simulink model "problem1"  (R2020b)
settings: Solver=VariableStepAuto  StartTime=0.0  StopTime=10.0  RelTol=1e-3
undefined symbols (not defined in the file): b, K1, K12, M1, M2
settings Model: Creator=admin  LastModifiedBy=admin

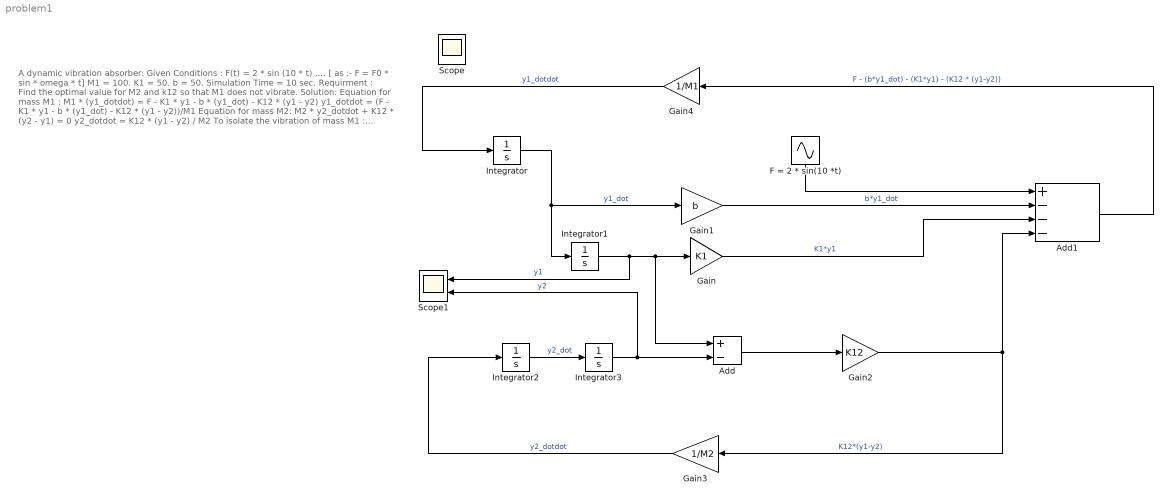
== system problem1 ==
  note: A dynamic vibration absorber:
      |
      | Given Conditions :
      | F(t) = 2 * sin (10 * t) .... [ as :- F = F0 * sin * omega * t]
      | M1 = 100. K1 = 50. b = 50.
      | Simulation Time = 10 sec.
      |
      | Requirment :
      | Find the optimal value for M2 and k12 so that M1 does not vibrate.
      |
      | Solution:
      | Equation for mass M1 :
      | M1 * (y1_dotdot) = F - K1 * y1 - b * (y1_dot) - K12 * (y1 - y2)
      |
      | y1_dotdot = (F - K1 * y1 - b * (y1_dot) - K12 * (y1 - y2))/M1
      |
      | Equation for mass M2:
      | M2 * y2_dotdot + K12 * (y2 - y1) = 0
      |
      | y2_dotdot = K12 * (y1 - y2) / M2
      |
      | To isolate the vibration of mass M1 :
      | usually, M1/M1 = (0.05 - 0.25)
  Add : Sum  Inputs=+-
  Add1 : Sum  Inputs=+---
  F = 2 * sin(10 *t) : Sin  Amplitude=2  Frequency=10  SampleTime=0
  Gain : Gain  Gain=K1
  Gain1 : Gain  Gain=b
  Gain2 : Gain  Gain=K12
  Gain3 : Gain  Gain=1/M2
  Gain4 : Gain  Gain=1/M1
  Integrator{,1..3} (4 alike) : Integrator
  Scope1 : Scope  NumInputPorts=2
  Scope : Scope
  wires:
  Integrator/1 -> Gain1/1, Integrator1/1  "y1_dot"
  Integrator1/1 -> Scope1/1, Add/1, Gain/1  "y1"
  Gain4/1 -> Integrator/1  "y1_dotdot"
  Integrator2/1 -> Integrator3/1  "y2_dot"
  Gain3/1 -> Integrator2/1  "y2_dotdot"
  Integrator3/1 -> Add/2, Scope1/2  "y2"
  Add/1 -> Gain2/1
  Gain/1 -> Add1/3  "K1*y1"
  Gain1/1 -> Add1/2  "b*y1_dot"
  Gain2/1 -> Gain3/1, Add1/4  "K12*(y1-y2)"
  F = 2 * sin(10 *t)/1 -> Add1/1
  Add1/1 -> Gain4/1  "F - (b*y1_dot) - (K1*y1) - (K12 * (y1-y2))"
